simulink model "sistema"  (R2025a)
settings: Solver=ode23t  StartTime=0.0  StopTime=10.0  MaxStep=1E-3  RelTol=1e-3
libraries: slpidlib x1, simulink x1
settings DataIOCC: ReturnWorkspaceOutputs=off  TimeSaveName=t
settings DebuggingCC: AlgebraicLoopMsg=none  ArtificialAlgebraicLoopMsg=none  MaxConsecutiveZCsMsg=none

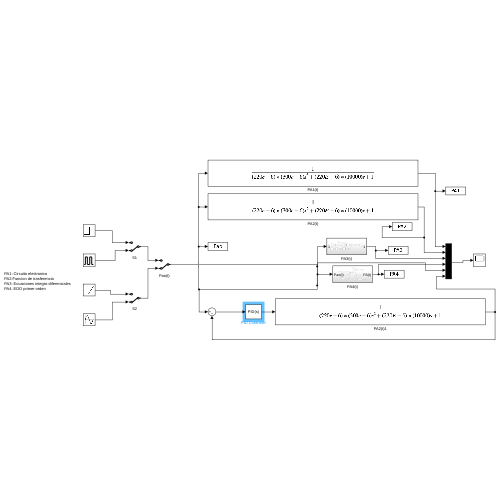
[thumbnail: Simulink's stored preview of the top-level diagram]
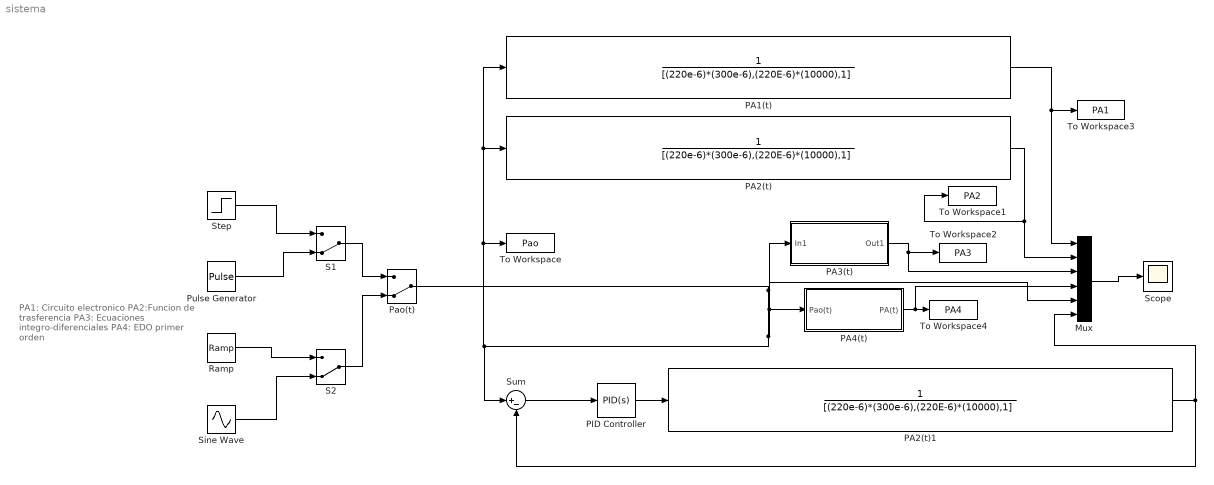
== system sistema ==
  note: PA1: Circuito electronico
      | PA2:Funcion de trasferencia
      | PA3: Ecuaciones integro-diferenciales
      | PA4: EDO primer orden
  Mux : Mux  Inputs=6
  PA1(t) : TransferFcn  Denominator=[(220e-6)*(300e-6),(220E-6)*(10000),1]
  PA2(t) : TransferFcn  Denominator=[(220e-6)*(300e-6),(220E-6)*(10000),1]
  PA2(t)1 : TransferFcn  Denominator=[(220e-6)*(300e-6),(220E-6)*(10000),1]
  PA3(t) : Subsystem
  PA4(t) : Subsystem
  PID Controller : slpidlib/PID Controller  Controller=PID  Form=Parallel  TimeDomain=Continuous-time  UseExternalTs=off  SampleTime=-1  IntegratorMethod=Forward Euler  FilterMethod=Forward Euler  ControllerParametersSource=internal  P=299.0263  I=7525.538  UseKiTs=off  D=0.39157  UseExternalDerivativeSource=off  N=519.2506  UseFilter=on  TunerSelectOption=Transfer Function Based (PID Tuner App)  InitialConditionSource=internal  InitialConditionForIntegrator=0  InitialConditionForFilter=0  DifferentiatorICPrevScaledInput=0  ExternalReset=none  TrackingMode=off  Kt=1  LimitOutput=off  SatLimitsSource=internal  UpperSaturationLimit=inf  LowerSaturationLimit=-inf  LinearizeAsGain=on  AntiWindupMode=none  Kb=1  LimitIntegrator=off  UpperIntegratorSaturationLimit=inf  LowerIntegratorSaturationLimit=-inf  POutMin=[]  POutMax=[]  IOutMin=[]  IOutMax=[]  DOutMin=[]  DOutMax=[]  NOutMin=[]  NOutMax=[]  SumOutMin=[]  SumOutMax=[]  SaturationOutMin=[]  SaturationOutMax=[]  PParamMin=[]  PParamMax=[]  IParamMin=[]  IParamMax=[]  DParamMin=[]  DParamMax=[]  NParamMin=[]  NParamMax=[]  KbParamMin=[]  KbParamMax=[]  KtParamMin=[]  KtParamMax=[]  KbOutMin=[]  KbOutMax=[]  KtOutMin=[]  KtOutMax=[]  IntegratorOutMin=[]  IntegratorOutMax=[]  FilterOutMin=[]  FilterOutMax=[]  SumI1OutMin=[]  SumI1OutMax=[]  SumI2OutMin=[]  SumI2OutMax=[]  SumI3OutMin=[]  SumI3OutMax=[]  SumI4OutMin=[]  SumI4OutMax=[]  SumDOutMin=[]  SumDOutMax=[]  DifferentiatorOutMin=[]  DifferentiatorOutMax=[]  FilterDiffOutCoefMin=[]  FilterDiffOutCoefMax=[]  ReciprocalOutMin=[]  ReciprocalOutMax=[]  SumDenOutMin=[]  SumDenOutMax=[]  SumNumOutMin=[]  SumNumOutMax=[]  DivideOutMin=[]  DivideOutMax=[]  UdiffTsProdOutMin=[]  UdiffTsProdOutMax=[]  NTsProdOutMin=[]  NTsProdOutMax=[]  UintegralTsProdOutMin=[]  UintegralTsProdOutMax=[]  UngainTsProdOutMin=[]  UngainTsProdOutMax=[]  ClampingZeroOutDataTypeStr=Inherit: Inherit via back propagation  ClampingZeroOutMin=[]  ClampingZeroOutMax=[]  FilterDenConstantOutDataTypeStr=Inherit: Inherit via back propagation  FilterDenConstantOutMin=[]  FilterDenConstantOutMax=[]  PCopyOutDataTypeStr=Inherit: Inherit via back propagation  PCopyOutMin=[]  PCopyOutMax=[]  NCopyOutDataTypeStr=Inherit: Inherit via back propagation  NCopyOutMin=[]  NCopyOutMax=[]  IntegratorContinuousStateAttributes=''  IntegratorStateMustResolveToSignalObject=off  IntegratorRTWStateStorageClass=Auto  FilterContinuousStateAttributes=''  FilterStateMustResolveToSignalObject=off  FilterRTWStateStorageClass=Auto  ParallelPVariant=InternalParameters  IdealPVariant=Disabled  IVariant=InternalParameters  DVariant=InternalParameters  IntegratorVariant=Continuous  SatVariant=Disabled  AWVariant=Passthrough  PCopyVariant=Disabled  TRVariant=Disabled  FdbkBlocksVariant=Forward  IdealPFdbkVariant=Disabled  SatFdbkVariant=Disabled  DerivativeFilterVariant=ContFilter  NVariant=InternalParameters  NCopyVariant=Disabled  FilterICVariant=InternalICsFilter  IntegratorICVariant=InternalICs  ExternalResetVariant=Disabled  TRSumVariant=Passthrough  SumFdbkVariant=Disabled  SumVariant=Sum_PID  TsampFilterVariant=InternalTs  TsampNgainVariant=Passthrough  TsampIntegralVariant=Disabled_SignalSpec  ExternalSaturationOutDataTypeStr=Inherit: Same as second input  DerivativeSourceVariant=ErrorSignal  PreIntVariant=InternalPreInt
  Pao(t) : ManualSwitch  CurrentSetting=0
  Pulse Generator : DiscretePulseGenerator  PulseType=Time based  Period=10  PulseWidth=10  PhaseDelay=1
  Ramp : simulink/Sources/Ramp  slope=1/10  start=0  InitialOutput=0
  S1 : ManualSwitch  CurrentSetting=0
  S2 : ManualSwitch  CurrentSetting=0
  Scope : Scope
      settings: ActiveDisplayYMinimum=-0.33856523116076365  ActiveDisplayYMaximum=1.2308990890400975
  Sine Wave : Sin  Frequency=pi/2  SampleTime=0
  Step : Step  Time=0  SampleTime=0.001
  Sum : Sum  Inputs=|+-
  To Workspace : ToWorkspace  VariableName=Pao  SampleTime=-1
  To Workspace1 : ToWorkspace  VariableName=PA2  SampleTime=-1
  To Workspace2 : ToWorkspace  VariableName=PA3  SampleTime=-1
  To Workspace3 : ToWorkspace  VariableName=PA1  SampleTime=-1
  To Workspace4 : ToWorkspace  VariableName=PA4  SampleTime=-1
  wires:
  Pulse Generator/1 -> S1/2
  Step/1 -> S1/1
  Ramp/1 -> S2/1
  Sine Wave/1 -> S2/2
  S2/1 -> Pao(t)/2
  S1/1 -> Pao(t)/1
  Pao(t)/1 -> PA3(t)/1(In1), Sum/1, To Workspace/1, PA1(t)/1, PA2(t)/1, Mux/5, PA4(t)/1(Pao(t))
  PA4(t)/1(PA(t)) -> Mux/4, To Workspace4/1
  PA3(t)/1(Out1) -> To Workspace2/1, Mux/3
  PA2(t)/1 -> Mux/2, To Workspace1/1
  Mux/1 -> Scope/1
  PA1(t)/1 -> To Workspace3/1, Mux/1
  Sum/1 -> PID Controller/1
  PID Controller/1 -> PA2(t)1/1
  PA2(t)1/1 -> Sum/2, Mux/6

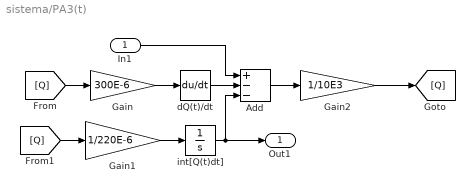
== system sistema/PA3(t) ==
  In1 : Inport
  Add : Sum  Inputs=+--
  Gain : Gain  Gain=300E-6
  Gain1 : Gain  Gain=1/220E-6
  Gain2 : Gain  Gain=1/10E3
  dQ(t)/dt : Derivative
  int[Q(t)dt] : Integrator
  Out1 : Outport
  wires:
  dQ(t)/dt/1 -> Add/2
  Add/1 -> Gain2/1
  int[Q(t)dt]/1 -> Out1/1, Add/3
  In1/1 -> Add/1
  [Q] -> Gain/1
  Gain/1 -> dQ(t)/dt/1
  Gain1/1 -> int[Q(t)dt]/1
  [Q] -> Gain1/1
  Gain2/1 -> [Q]

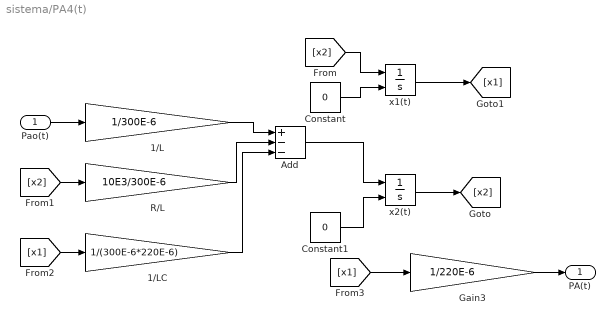
== system sistema/PA4(t) ==
  Pao(t) : Inport
  1/L : Gain  Gain=1/300E-6
  1/LC : Gain  Gain=1/(300E-6*220E-6)
  Add : Sum  Inputs=+--
  Constant : Constant  Value=0
  Constant1 : Constant  Value=0
  Gain3 : Gain  Gain=1/220E-6
  R/L : Gain  Gain=10E3/300E-6
  x1(t) : Integrator  InitialConditionSource=external
  x2(t) : Integrator  InitialConditionSource=external
  PA(t) : Outport
  wires:
  Constant/1 -> x1(t)/2
  Constant1/1 -> x2(t)/2
  x1(t)/1 -> [x1]
  [x2] -> x1(t)/1
  x2(t)/1 -> [x2]
  Add/1 -> x2(t)/1
  1/L/1 -> Add/1
  Pao(t)/1 -> 1/L/1
  [x2] -> R/L/1
  R/L/1 -> Add/2
  [x1] -> 1/LC/1
  1/LC/1 -> Add/3
  [x1] -> Gain3/1
  Gain3/1 -> PA(t)/1
